simulink model "LSE_csi"  (R2016b)
settings: Solver=VariableStepAuto  StartTime=0.0  StopTime=10.0  RelTol=1e-3
settings Model: Creator=CHAITRA  LastModifiedBy=CHAITRA

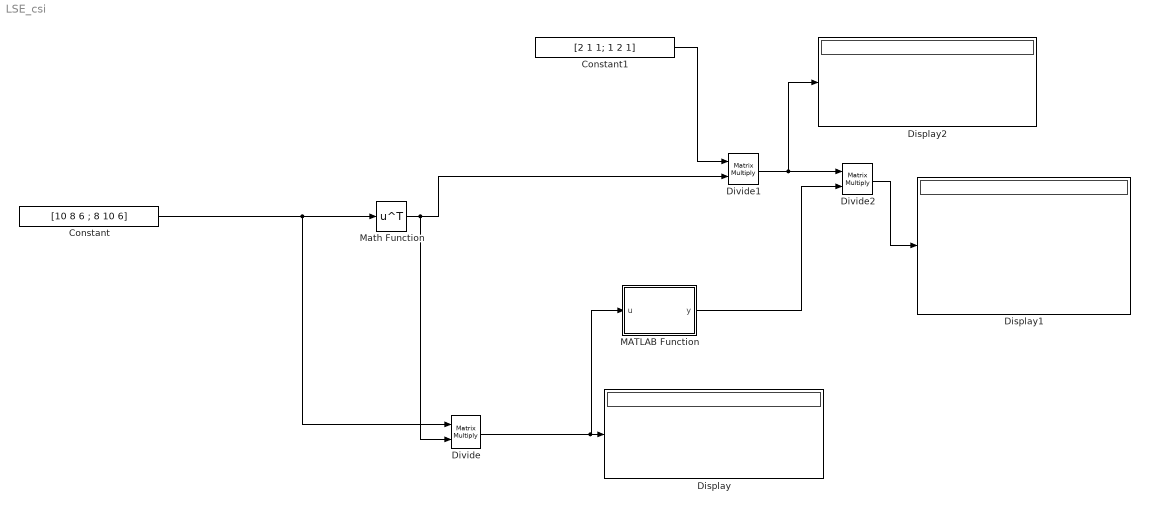
== system LSE_csi ==
  Constant : Constant  Value=[10 8 6 ; 8 10 6]
  Constant1 : Constant  Value=[2 1 1; 1 2 1]
  Display : Display
  Display1 : Display
  Display2 : Display
  Divide : Product  Multiplication=Matrix(*)
  Divide1 : Product  Multiplication=Matrix(*)
  Divide2 : Product  Multiplication=Matrix(*)
  MATLAB Function : MATLAB Function  TreatAsAtomicUnit=on
  Math Function : Math  Operator=transpose  SaturateOnIntegerOverflow=on
  wires:
  Math Function/1 -> Divide/2, Divide1/2
  Divide/1 -> MATLAB Function/1(u), Display/1
  MATLAB Function/1(y) -> Divide2/2
  Divide1/1 -> Display2/1, Divide2/1
  Divide2/1 -> Display1/1
  Constant/1 -> Divide/1, Math Function/1
  Constant1/1 -> Divide1/1

== matlab function LSE_csi/MATLAB Function ==
  data: u input; y output
function y = fcn(u)

y = inv(u);
